simulink model "ball_animation"  (Simulink 8.3)
settings: Solver=ode45  StartTime=0.0  StopTime=10000  RelTol=1e-3
undefined symbols (not defined in the file or in its folder): drawBall
libraries: simulink x2
settings Model: Creator=beard  LastModifiedBy=jhl48
settings OptimizationCC: ExpressionDepthLimit=2147483647  InitFltsAndDblsToZero=on
settings DebuggingCC: FcnCallInpInsideContextMsg=UseLocalSettings

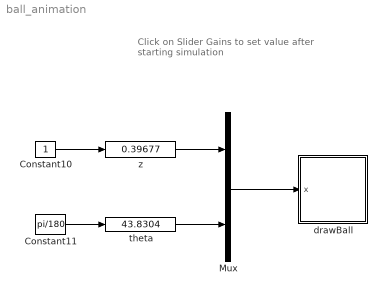
== system ball_animation ==
  note: Click on Slider Gains to set value
      | after starting simulation
  Constant10 : Constant
  Constant11 : Constant  Value=pi/180
  Mux : Mux  Inputs=2
  drawBall : Subsystem
      mask init:
      | % drawing parameters
      | L = 1;
      | gap = 0.01;
      | width = 1.0;
      | height = 0.1;
      mask Display: image(imread('tv.jpg'))
  theta : simulink/Math Operations/Slider Gain  low=-180  gain=43.8304  high=180
  z : simulink/Math Operations/Slider Gain  low=-3  gain=0.39677  high=3
  wires:
  z/1 -> Mux/1
  Constant10/1 -> z/1
  theta/1 -> Mux/2
  Constant11/1 -> theta/1
  Mux/1 -> drawBall/1(x)

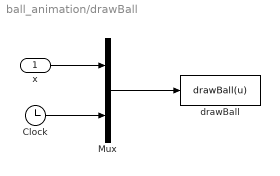
== system ball_animation/drawBall ==
  x : Inport
  Clock : Clock
  Mux : Mux  Inputs=2
  drawBall : MATLABFcn  MATLABFcn=drawBall(u)  OutputDimensions=0  SampleTime=0.1
  wires:
  Mux/1 -> drawBall/1
  x/1 -> Mux/1
  Clock/1 -> Mux/2
